simulink model "detectPerson"  (R2016a)
settings: Solver=FixedStepAuto  StartTime=0.0  StopTime=inf  FixedStep=0.01  RelTol=1e-3
InitFcn:
  | data_len = 63504+16;
libraries: visiontextngfix x3, visionsinks x1, visiongeotforms x1, dspnetwork x1
settings Model: ModifiedByFormat=mbd_app  Creator=mbd_app  LastModifiedBy=mbd_app
settings DataIOCC: SaveOutput=off  SignalLogging=off  DSMLogging=off  SaveTime=off

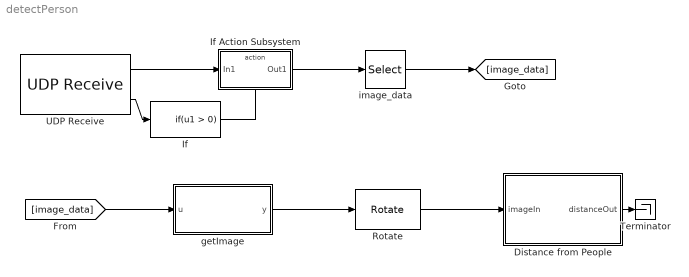
== system detectPerson ==
  Distance from People : Subsystem
  If : If  ShowElse=off
  If Action Subsystem : Subsystem  TreatAsAtomicUnit=on
  Rotate : visiongeotforms/Rotate  outSizeR=Expanded to fit rotated input image  src_angle=Specify via dialog  unit_angle=Degrees  angle=pi/2  maxAngle=pi  dispImage=Center  method=Table lookup  fillVal=0  interpMethod=Bilinear  prodOutputMode=Binary point scaling  prodOutputWordLength=32  prodOutputFracLength=10  roundingMode=Nearest  overflowMode=on
  Terminator : Terminator
  UDP Receive : dspnetwork/UDP Receive  localURL='0.0.0.0'  localPort=8027  remoteURL='0.0.0.0'  remotePort=-1  recvBufferSize=65300  dims=data_len  signalDatatype=uint8  isVarSize=off  showBlockingTime=on  blockingTime=1  sampletime=1  blockPlatform=HOST
  getImage : MATLAB Function  TreatAsAtomicUnit=on
  image_data : Selector  InputPortWidth=data_len  IndexOptions=Index vector (dialog)  Indices=17:data_len  OutputSizes=1
  wires:
  If Action Subsystem/1(Out1) -> image_data/1
  UDP Receive/2 -> If/1
  image_data/1 -> [image_data]
  getImage/1(y) -> Rotate/1
  Rotate/1 -> Distance from People/1(imageIn)
  UDP Receive/1 -> If Action Subsystem/1(In1)
  If/1 -> If Action Subsystem/Action
  [image_data] -> getImage/1(u)
  Distance from People/1(distanceOut) -> Terminator/1

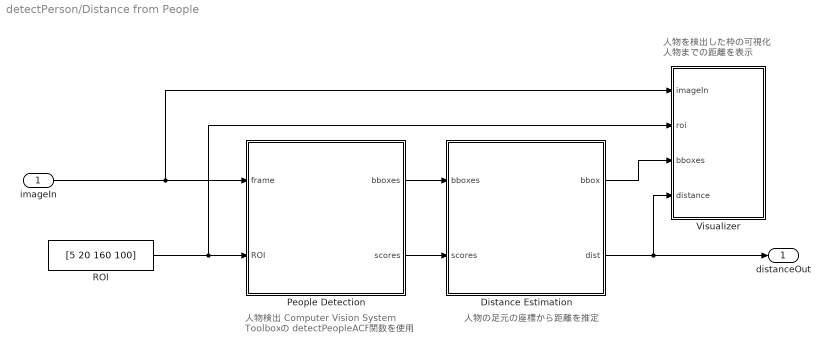
== system detectPerson/Distance from People ==
  note: 人物検出
      | Computer Vision System Toolboxの
      | detectPeopleACF関数を使用
  note: 人物の足元の座標から距離を推定
  note: 人物を検出した枠の可視化
      | 人物までの距離を表示
  imageIn : Inport
  Distance Estimation : MATLAB Function  TreatAsAtomicUnit=on
  People Detection : MATLAB Function  TreatAsAtomicUnit=on
  ROI : Constant  Value=[5 20 160 100]
  Visualizer : Subsystem
  distanceOut : Outport
  wires:
  imageIn/1 -> Visualizer/1(imageIn), People Detection/1(frame)
  People Detection/2(scores) -> Distance Estimation/2(scores)
  People Detection/1(bboxes) -> Distance Estimation/1(bboxes)
  Distance Estimation/1(bbox) -> Visualizer/3(bboxes)
  Distance Estimation/2(dist) -> distanceOut/1, Visualizer/4(distance)
  ROI/1 -> Visualizer/2(roi), People Detection/2(ROI)

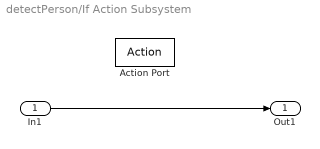
== system detectPerson/If Action Subsystem ==
  In1 : Inport
  Action Port : ActionPort  ActionType=then
  Out1 : Outport
  wires:
  In1/1 -> Out1/1

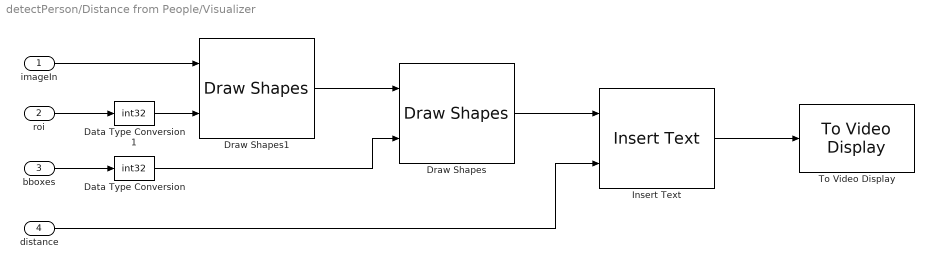
== system detectPerson/Distance from People/Visualizer ==
  imageIn : Inport
  roi : Inport  Port=2
  bboxes : Inport  Port=3
  distance : Inport  Port=4
  Data Type Conversion : DataTypeConversion  OutDataTypeStr=int32
  Data Type Conversion1 : DataTypeConversion  OutDataTypeStr=int32
  Draw Shapes : visiontextngfix/Draw Shapes  shape=Rectangles  fill=off  lineWidth=3  fillClrSource=Specify via dialog  display=User-specified value  intensity=200  color=[255 0 0]  opacity=0.6  viewport=Entire image  antialiasing=off  inType=Obsolete  imagePorts=One multidimensional signal  prodOutputMode=Binary point scaling  prodOutputWordLength=32  prodOutputFracLength=14  memoryMode=Specify word length  memoryWordLength=16  memoryFracLength=15  roundingMode=Floor  overflowMode=off
  Draw Shapes1 : visiontextngfix/Draw Shapes  shape=Rectangles  fill=off  lineWidth=3  fillClrSource=Specify via dialog  display=User-specified value  intensity=200  color=[255 0 255]  opacity=0.6  viewport=Entire image  antialiasing=off  inType=Obsolete  imagePorts=One multidimensional signal  prodOutputMode=Binary point scaling  prodOutputWordLength=32  prodOutputFracLength=14  memoryMode=Specify word length  memoryWordLength=16  memoryFracLength=15  roundingMode=Floor  overflowMode=off
  Insert Text : visiontextngfix/Insert Text  inputType=Obsolete  theText='Estimated distance = %.1fm'  getTextLocFrom=Specify via dialog  textLoc=[1 1]  getTextColorFrom=Specify via dialog  textColor=[255 0 0]  getTextIntensityFrom=Specify via dialog  textIntensity=0  getTextOpacityFrom=Specify via dialog  textOpacity=1.0  dummyVar2=0  dummyVar3=0  dummyVar4=0  imagePorts=One multidimensional signal  isInputTransposed=off  fontFace=LucidaSansRegular  dummyVar1=0  blockFontSize=12  antiAliased=on
  To Video Display : visionsinks/To Video Display  windowSizeMode=Normal  openAtMdlStart=on  fullScreen=off  videoWindowX=1336  videoWindowY=156  saveWindowSize=off  videoWindowWidth=343  videoWindowHeight=252  inputColorFormat=RGB  inputType=Obsolete  imagePorts=One multidimensional signal  OutputDevice=On-screen video monitor  dataOrg=Column-major  isWindowOpen=off
  wires:
  Data Type Conversion1/1 -> Draw Shapes1/2
  Draw Shapes1/1 -> Draw Shapes/1
  roi/1 -> Data Type Conversion1/1
  Data Type Conversion/1 -> Draw Shapes/2
  distance/1 -> Insert Text/2
  bboxes/1 -> Data Type Conversion/1
  imageIn/1 -> Draw Shapes1/1
  Draw Shapes/1 -> Insert Text/1
  Insert Text/1 -> To Video Display/1

== matlab function detectPerson/getImage ==
  data: u input uint8; y output uint8
function y = fcn(u)
%#codegen
w = 168;
h = 126;

y = uint8(zeros(w, h, 3));

temp = reshape(u, 3, length(u)/3);

y(:, :, 1) = reshape(temp(1, :), w, h);
y(:, :, 2) = reshape(temp(2, :), w, h);
y(:, :, 3) = reshape(temp(3, :), w, h);

% [EOF]

== matlab function detectPerson/Distance from People/Distance Estimation ==
  data: bbox output; bboxes input size=[100 4]; scores input size=[100 1]; dist output
function [bbox,dist] = estimateDistance(bboxes,scores)
if isempty(bboxes)
    dist = 0;
    bbox = [0 0 0 0];
else
    [~,indMax] = max(scores); % 一番、人物らしい枠を抽出
    bbox = bboxes(indMax,1:4); % バウンディングボックスを抽出
    height = bbox(1, 4); % 高さを取得
    dist = 100/height; % 人の高さが一定として距離を計算
end

== matlab function detectPerson/Distance from People/People Detection ==
  data: bboxes output size=[100 4]; frame input; ROI input size=[1 4]; scores output size=[100 1]
function [bboxes, scores] = detectPeople(frame,ROI)
%#codegen
coder.extrinsic('detectPeopleACF');
bboxes = zeros(100,4); %#ok<*PREALL>
scores = zeros(100,1);

% Computer Vision System Toolboxの人物検出の関数を使用
[bboxes,scores] = detectPeopleACF(frame, ROI, ...
            'Model','caltech',...
            'WindowStride', 2,...
            'NumScaleLevels', 4, ...
            'SelectStrongest', false);

% [EOF]
